simulink model "controlSystem_TorqueOptimizer"  (R2021a)
settings: Solver=VariableStepAuto  StartTime=0.0  StopTime=30  RelTol=1e-7
values from neighbouring files (symbols this model uses):
  initialFuel = 100    [data.m]
  maxEngineTemp = 240    [data.m]
  maxEngineTorque = 80    [data.m]
  maxMotorTemp = 135    [data.m]
  maxMotorTorque = 80    [data.m]
  maxRegenTorque = 80    [data.m]
  motorVoltage = 140    [data.m]
undefined symbols (not defined in the file or in its folder): sigbuilder_block
libraries: autolibshared x4, autolibsharedcoupling x3, autolibhevctrlrcommon x2, autolibmappedmotor x2, autolibshareddiff x1, autolibtransamt x1, autolibdcdc x1, autolibdatasheetbattery x1, autolibsharedmappedengines x1
(part 5 of 5)

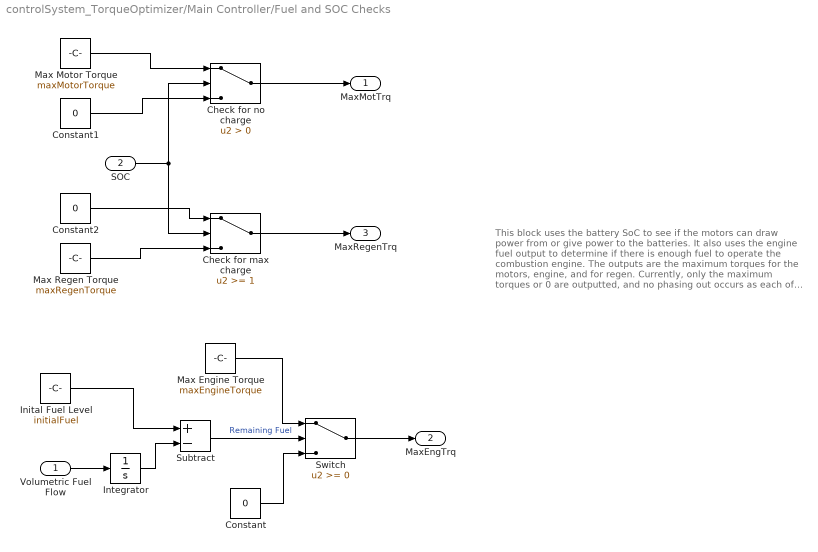
== system controlSystem_TorqueOptimizer/Main Controller/Fuel and SOC Checks ==
  note: This block uses the battery SoC to see if the motors can draw power from or give power to the batteries. It also uses the engine fuel output to determine if there is enough fuel to operate the combustion engine. The outputs are the maximum torques for the motors, engine, and for regen.
      |
      | Currently, only the maximum torques or 0 are outputted, and no phasing out occurs as each of the power supply decreases.
  Volumetric Fuel Flow : Inport
  SOC : Inport  Port=2
  Check for max charge : Switch  Threshold=1
  Check for no charge : Switch  Criteria=u2 > Threshold
  Constant : Constant  Value=0
  Constant1 : Constant  Value=0
  Constant2 : Constant  Value=0
  Inital Fuel Level : Constant  Value=initialFuel
  Integrator : Integrator
  Max Engine Torque : Constant  Value=maxEngineTorque
  Max Motor Torque : Constant  Value=maxMotorTorque
  Max Regen Torque : Constant  Value=maxRegenTorque
  Subtract : Sum  Inputs=+-
  Switch : Switch
  MaxMotTrq : Outport
  MaxEngTrq : Outport  Port=2
  MaxRegenTrq : Outport  Port=3
  wires:
  Subtract/1 -> Switch/2  "Remaining Fuel"
  Constant/1 -> Switch/3
  Inital Fuel Level/1 -> Subtract/1
  Integrator/1 -> Subtract/2
  Volumetric Fuel Flow/1 -> Integrator/1
  Max Engine Torque/1 -> Switch/1
  Switch/1 -> MaxEngTrq/1
  Check for no charge/1 -> MaxMotTrq/1
  Check for max charge/1 -> MaxRegenTrq/1
  Max Motor Torque/1 -> Check for no charge/1
  Constant1/1 -> Check for no charge/3
  SOC/1 -> Check for max charge/2, Check for no charge/2
  Max Regen Torque/1 -> Check for max charge/3
  Constant2/1 -> Check for max charge/1

== system controlSystem_TorqueOptimizer/Main Controller/Heat Controller ==
  note: Decreases the torque to the motor or engine if they are overheating by the power of the stand-in gain function.
      | This system doesn't make the other motor/engine work harder if one is too hot. Therefore when one is overheated the car instantly loses power, instead of when both are overheated.
  Motor Torque : Inport
  Engine Torque : Inport  Port=2
  Engine Temp Switch : Switch  Criteria=u2 > Threshold  Threshold=maxEngineTemp
  Motor Temp Switch : Switch  Criteria=u2 > Threshold  Threshold=maxMotorTemp
  Signal Builder : Subsystem  Tag=STV Subsys  LoadFcn=sigbuilder_block('load');  StartFcn=sigbuilder_block('start');  StopFcn=sigbuilder_block('stop');  ClipboardFcn=sigbuilder_block('clipboard');  mask(Sigbuilder block){tuvar=[0:10]}
      mask help: Simulink:masks:SigbuilderBlock_MD
      mask init:
      | if ~strcmp(get_param(bdroot(gcbh),'SimulationStatus'),'stopped') tuvar = sigbuilder_block('maskInit'); end
      settings: CopyFcn=sigbuilder_block('copy');  DeleteFcn=sigbuilder_block('delete');  ModelCloseFcn=sigbuilder_block('modelClose');  PreSaveFcn=sigbuilder_block('preSave');  PauseFcn=sigbuilder_block('pause');  ContinueFcn=sigbuilder_block('continue');  NameChangeFcn=sigbuilder_block('namechange');  OpenFcn=sigbuilder_block('open',[411 128.5 543.5 351.5 ]);  CloseFcn=sigbuilder_block('close');
      mask Display: plot(0, 0, 100, 100,[2, 2, 32, 32, 2], [68, 8, 8, 68, 68],[32, 2], [38, 38], [32, 19, 2],[53, 60, 44], [32, 17, 17, 2],[16, 16, 31, 31]);txt = getActiveGroup(gcbh);text(2, 100, txt,'verticalAlignment', 'top');
  place-holder to decrease engine torque : Gain
  place-holder to decrease motor torque : Gain
  Updated Motor Torque : Outport
  Updated Engine Torque : Outport  Port=2
  wires:
  Motor Torque/1 -> place-holder to decrease motor torque/1, Motor Temp Switch/3
  place-holder to decrease motor torque/1 -> Motor Temp Switch/1
  Engine Torque/1 -> place-holder to decrease engine torque/1, Engine Temp Switch/3
  place-holder to decrease engine torque/1 -> Engine Temp Switch/1
  Signal Builder/1(Motor temp) -> Motor Temp Switch/2
  Signal Builder/2(Engine temp) -> Engine Temp Switch/2
  Motor Temp Switch/1 -> Updated Motor Torque/1
  Engine Temp Switch/1 -> Updated Engine Torque/1

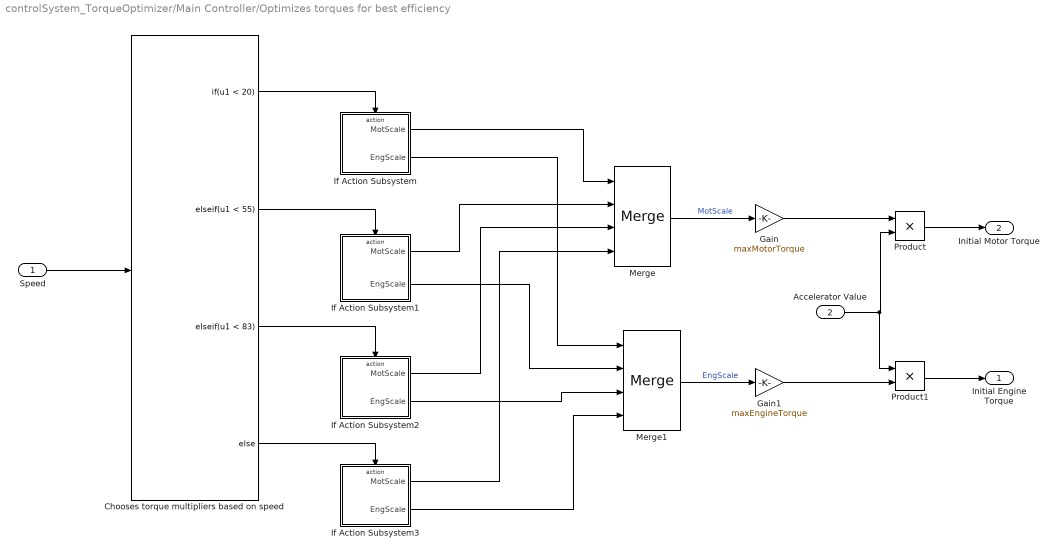
== system controlSystem_TorqueOptimizer/Main Controller/Optimizes torques for best efficiency ==
  Speed : Inport
  Accelerator Value : Inport  Port=2
  Chooses torque multipliers based on speed : If  IfExpression=u1 < 20  ElseIfExpressions=u1 < 55, u1 < 83
  Gain : Gain  Gain=maxMotorTorque
  Gain1 : Gain  Gain=maxEngineTorque
  If Action Subsystem : Subsystem  TreatAsAtomicUnit=on
  If Action Subsystem1 : Subsystem  TreatAsAtomicUnit=on
  If Action Subsystem2 : Subsystem  TreatAsAtomicUnit=on
  If Action Subsystem3 : Subsystem  TreatAsAtomicUnit=on
  Merge : Merge  Inputs=4
  Merge1 : Merge  Inputs=4
  Product : Product
  Product1 : Product
  Initial Engine Torque : Outport
  Initial Motor Torque : Outport  Port=2
  wires:
  Speed/1 -> Chooses torque multipliers based on speed/1
  Chooses torque multipliers based on speed/1 -> If Action Subsystem/Action
  Chooses torque multipliers based on speed/4 -> If Action Subsystem3/Action
  Chooses torque multipliers based on speed/3 -> If Action Subsystem2/Action
  Chooses torque multipliers based on speed/2 -> If Action Subsystem1/Action
  If Action Subsystem/1(MotScale) -> Merge/1
  If Action Subsystem1/1(MotScale) -> Merge/2
  If Action Subsystem2/1(MotScale) -> Merge/3
  If Action Subsystem3/1(MotScale) -> Merge/4
  If Action Subsystem/2(EngScale) -> Merge1/1
  If Action Subsystem1/2(EngScale) -> Merge1/2
  If Action Subsystem2/2(EngScale) -> Merge1/3
  If Action Subsystem3/2(EngScale) -> Merge1/4
  Merge1/1 -> Gain1/1  "EngScale"
  Merge/1 -> Gain/1  "MotScale"
  Accelerator Value/1 -> Product1/1, Product/2
  Product1/1 -> Initial Engine Torque/1
  Product/1 -> Initial Motor Torque/1
  Gain1/1 -> Product1/2
  Gain/1 -> Product/1

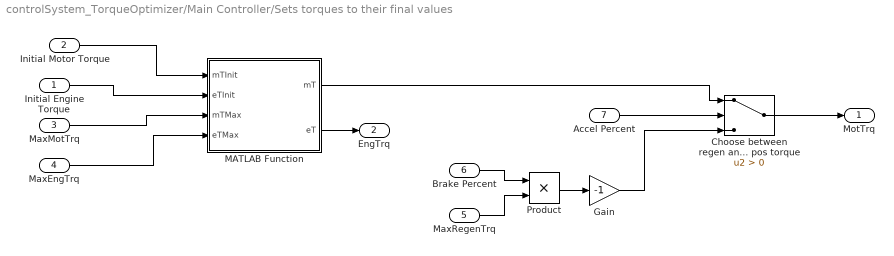
== system controlSystem_TorqueOptimizer/Main Controller/Sets torques to their final values ==
  Initial Engine Torque : Inport
  Initial Motor Torque : Inport  Port=2
  MaxMotTrq : Inport  Port=3
  MaxEngTrq : Inport  Port=4
  MaxRegenTrq : Inport  Port=5
  Brake Percent : Inport  Port=6
  Accel Percent : Inport  Port=7
  Choose between regen and pos torque : Switch  Criteria=u2 > Threshold
  Gain : Gain  Gain=-1
  MATLAB Function : MATLAB Function  TreatAsAtomicUnit=on
  Product : Product
  MotTrq : Outport
  EngTrq : Outport  Port=2
  wires:
  Gain/1 -> Choose between regen and pos torque/3
  MaxMotTrq/1 -> MATLAB Function/3(mTMax)
  MaxEngTrq/1 -> MATLAB Function/4(eTMax)
  Product/1 -> Gain/1
  Choose between regen and pos torque/1 -> MotTrq/1
  Brake Percent/1 -> Product/1
  Accel Percent/1 -> Choose between regen and pos torque/2
  MaxRegenTrq/1 -> Product/2
  Initial Motor Torque/1 -> MATLAB Function/1(mTInit)
  Initial Engine Torque/1 -> MATLAB Function/2(eTInit)
  MATLAB Function/2(eT) -> EngTrq/1
  MATLAB Function/1(mT) -> Choose between regen and pos torque/1

== system controlSystem_TorqueOptimizer/SI Engine/Accessory Load Model ==
  EngTrqIn : Inport
  EngSpd : Inport  Port=2
  Accessory Load Model : autolibhevctrlrcommon/Accessory Load Model  AccPwrTbl=[0 0]  AccSpdBpts=[300 750]
      settings: SourceProductBaseCode=PW
  Lumped Torque Dynamics : TransferFcn  Denominator=[0.2 1]
  Net Torque : Sum  Inputs=+-
  EngTrqOut : Outport  Unit=N*m  VectorParamsAs1DForOutWhenUnconnected=off
  wires:
  EngSpd/1 -> Accessory Load Model/1
  Lumped Torque Dynamics/1 -> EngTrqOut/1
  Net Torque/1 -> Lumped Torque Dynamics/1
  EngTrqIn/1 -> Net Torque/1
  Accessory Load Model/1 -> Net Torque/2

== system controlSystem_TorqueOptimizer/Drivetrain/Transmission/Accessory Load Model ==
  EngTrqIn : Inport
  EngSpd : Inport  Port=2
  Accessory Load Model : autolibhevctrlrcommon/Accessory Load Model  AccPwrTbl=[0 0]  AccSpdBpts=[300 750]
      settings: SourceProductBaseCode=PW
  Lumped Torque Dynamics : TransferFcn  Denominator=[0.2 1]
  Net Torque : Sum  Inputs=+-
  EngTrqOut : Outport  Unit=N*m  VectorParamsAs1DForOutWhenUnconnected=off
  wires:
  EngSpd/1 -> Accessory Load Model/1
  Lumped Torque Dynamics/1 -> EngTrqOut/1
  Net Torque/1 -> Lumped Torque Dynamics/1
  EngTrqIn/1 -> Net Torque/1
  Accessory Load Model/1 -> Net Torque/2

== system controlSystem_TorqueOptimizer/Drivetrain/Transmission/Subsystem ==
  note: Gear Selection based on current vehicle speed
  VehSpdFdbk : Inport
  Gear 1 : Subsystem  TreatAsAtomicUnit=on
  Gear 2 : Subsystem  TreatAsAtomicUnit=on
  Gear 3 : Subsystem  TreatAsAtomicUnit=on
  Gear 4 : Subsystem  TreatAsAtomicUnit=on
  Gear 6 : Subsystem  TreatAsAtomicUnit=on
  Gear Chooser : If  IfExpression=u1 < 49.31  ElseIfExpressions=u1 < 60.69, u1 < 73.70, u1 < 88.70
  Selected Gear Merger : Merge  Inputs=5
  Gear : Outport
  wires:
  VehSpdFdbk/1 -> Gear Chooser/1
  Gear Chooser/1 -> Gear 1/Action
  Gear Chooser/2 -> Gear 2/Action
  Gear Chooser/3 -> Gear 3/Action
  Gear Chooser/4 -> Gear 4/Action
  Gear Chooser/5 -> Gear 6/Action
  Selected Gear Merger/1 -> Gear/1
  Gear 1/1(Out1) -> Selected Gear Merger/1
  Gear 2/1(Out1) -> Selected Gear Merger/2
  Gear 3/1(Out1) -> Selected Gear Merger/3
  Gear 4/1(Out1) -> Selected Gear Merger/4
  Gear 6/1(Out1) -> Selected Gear Merger/5

== system controlSystem_TorqueOptimizer/Main Controller/Heat Controller/Signal Builder ==
  Demux : Demux  Tag=STV Demux  Outputs=2
      settings: DisplayOption=none
  FromWs : FromWorkspace  Tag=STV FromWs  VariableName=tuvar
      SigBuilderData=|
      | common.afterFinalStr = 'Extrapolate'
      | common.sampleTime = 0
      | dataSet.timeRange = [0 10]
      | dataSet.name = 'Temperature Signals'
      | sbobj.Groups.Name = 'Temperature Signals'
      | sbobj.Groups.Signals(1).Name = 'Motor temp'
      | sbobj.Groups.Signals(1).XData = [0 10]
      | sbobj.Groups.Signals(1).YData = [0 0]
      | sbobj.Groups.Signals(2).Name = 'Engine temp'
      | sbobj.Groups.Signals(2).XData = [0 10]
      | sbobj.Groups.Signals(2).YData = [0 0]
  Motor temp : Outport  Tag=STV Outport
  Engine temp : Outport  Tag=STV Outport  Port=2
  wires:
  FromWs/1 -> Demux/1
  Demux/1 -> Motor temp/1
  Demux/2 -> Engine temp/1

== system controlSystem_TorqueOptimizer/Main Controller/Optimizes torques for best efficiency/If Action Subsystem ==
  Action Port : ActionPort  ActionPortLabel=if(u1 < 20)
  Constant : Constant
  Constant1 : Constant  Value=0
  MotScale : Outport
  EngScale : Outport  Port=2
  wires:
  Constant/1 -> MotScale/1
  Constant1/1 -> EngScale/1

== system controlSystem_TorqueOptimizer/Main Controller/Optimizes torques for best efficiency/If Action Subsystem1 ==
  Action Port : ActionPort  ActionPortLabel=elseif(u1 < 55)
  Constant : Constant  Value=0.6
  Constant1 : Constant  Value=0.4
  MotScale : Outport
  EngScale : Outport  Port=2
  wires:
  Constant/1 -> MotScale/1
  Constant1/1 -> EngScale/1

== system controlSystem_TorqueOptimizer/Main Controller/Optimizes torques for best efficiency/If Action Subsystem2 ==
  Action Port : ActionPort  ActionPortLabel=elseif( u1 < 83)
  Constant : Constant  Value=0.2
  Constant1 : Constant  Value=0.8
  MotScale : Outport
  EngScale : Outport  Port=2
  wires:
  Constant1/1 -> EngScale/1
  Constant/1 -> MotScale/1

== system controlSystem_TorqueOptimizer/Main Controller/Optimizes torques for best efficiency/If Action Subsystem3 ==
  Action Port : ActionPort  ActionPortLabel=else
  Constant : Constant  Value=0
  Constant1 : Constant
  MotScale : Outport
  EngScale : Outport  Port=2
  wires:
  Constant1/1 -> EngScale/1
  Constant/1 -> MotScale/1

== system controlSystem_TorqueOptimizer/Drivetrain/Transmission/Subsystem/Gear 1 ==
  Action Port : ActionPort  ActionPortLabel=if(u1 < 49.31)
  Constant : Constant
  Out1 : Outport
  wires:
  Constant/1 -> Out1/1

== system controlSystem_TorqueOptimizer/Drivetrain/Transmission/Subsystem/Gear 2 ==
  Action Port : ActionPort  ActionPortLabel=elseif(u1 < 60.69)
  Constant : Constant  Value=2
  Out1 : Outport
  wires:
  Constant/1 -> Out1/1

== system controlSystem_TorqueOptimizer/Drivetrain/Transmission/Subsystem/Gear 3 ==
  Action Port : ActionPort  ActionPortLabel=elseif( u1 < 73.70)
  Constant : Constant  Value=3
  Out1 : Outport
  wires:
  Constant/1 -> Out1/1

== system controlSystem_TorqueOptimizer/Drivetrain/Transmission/Subsystem/Gear 4 ==
  Action Port : ActionPort  ActionPortLabel=elseif( u1 < 88.70)
  Constant : Constant  Value=4
  Out1 : Outport
  wires:
  Constant/1 -> Out1/1

== system controlSystem_TorqueOptimizer/Drivetrain/Transmission/Subsystem/Gear 6 ==
  Action Port : ActionPort  ActionPortLabel=else
  Constant : Constant  Value=5
  Out1 : Outport
  wires:
  Constant/1 -> Out1/1

== matlab function controlSystem_TorqueOptimizer/Main Controller/Sets torques to their final values/MATLAB Function ==
  data: mTInit input; mT output; eTInit input; mTMax input; eTMax input; eT output
function [mT, eT] = fcn(mTInit, eTInit, mTMax, eTMax)
if (mTInit <= mTMax && eTInit <= eTMax) % both initial supplies are valid
    mT = mTInit;
    eT = eTInit;
elseif (mTInit > mTMax && eTInit <= eTMax) % motor torque is too high
    mT = mTMax;
    engSpace = (eTMax - eTInit);
    motOver = (mTInit - mTMax);
    if (engSpace > motOver) 
        eT = eTInit + motOver;
    else
        eT = eTMax;
    end
elseif (mTInit <= mTMax && eTInit > eTMax) % engine torue is too high
    eT = eTMax;
    motSpace = (mTMax - mTInit);
    engOver = (eTInit - eTMax);
    if (motSpace > engOver) 
        mT = mTInit + engOver;
    else
        mT = mTMax;
    end
else % both torques are too high
    mT = mTMax;
    eT = eTMax;
end
end
